simulink subsystem "Init_Frenet_Value"  (R2022b)
settings: Solver=VariableStepAuto  StartTime=0.0  StopTime=10.0  RelTol=1e-3
settings Model: Creator=User  LastModifiedBy=User

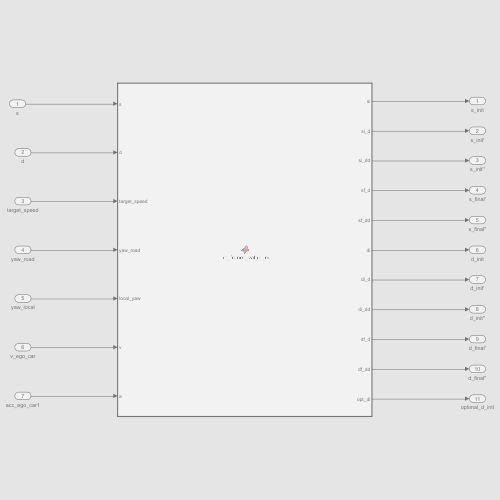
[thumbnail: Simulink's stored preview of the top-level diagram]
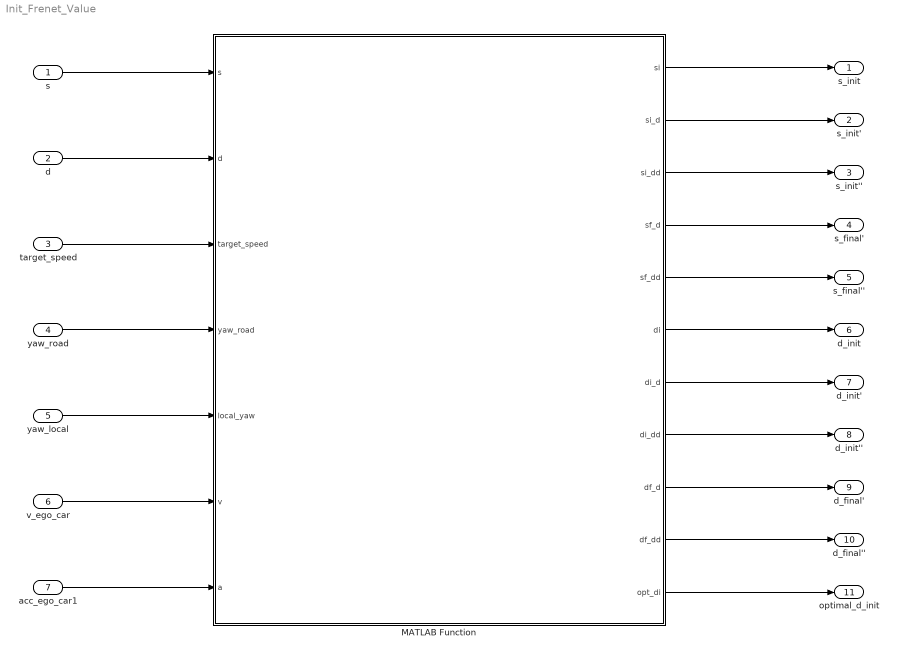
== system Init_Frenet_Value ==
  s : Inport
  d : Inport  Port=2
  target_speed : Inport  Port=3
  yaw_road : Inport  Port=4
  yaw_local : Inport  Port=5
  v_ego_car : Inport  Port=6
  acc_ego_car1 : Inport  Port=7
  MATLAB Function : MATLAB Function  TreatAsAtomicUnit=on
  s_init : Outport
  s_init' : Outport  Port=2
  s_init'' : Outport  Port=3
  s_final' : Outport  Port=4
  s_final'' : Outport  Port=5
  d_init : Outport  Port=6
  d_init' : Outport  Port=7
  d_init'' : Outport  Port=8
  d_final' : Outport  Port=9
  d_final'' : Outport  Port=10
  optimal_d_init : Outport  Port=11
  wires:
  acc_ego_car1/1 -> MATLAB Function/7(a)
  v_ego_car/1 -> MATLAB Function/6(v)
  yaw_local/1 -> MATLAB Function/5(local_yaw)
  MATLAB Function/11(opt_di) -> optimal_d_init/1
  MATLAB Function/10(df_dd) -> d_final''/1
  MATLAB Function/9(df_d) -> d_final'/1
  MATLAB Function/8(di_dd) -> d_init''/1
  MATLAB Function/7(di_d) -> d_init'/1
  MATLAB Function/6(di) -> d_init/1
  MATLAB Function/5(sf_dd) -> s_final''/1
  MATLAB Function/4(sf_d) -> s_final'/1
  MATLAB Function/3(si_dd) -> s_init''/1
  MATLAB Function/2(si_d) -> s_init'/1
  MATLAB Function/1(si) -> s_init/1
  target_speed/1 -> MATLAB Function/3(target_speed)
  yaw_road/1 -> MATLAB Function/4(yaw_road)
  d/1 -> MATLAB Function/2(d)
  s/1 -> MATLAB Function/1(s)

== matlab function Init_Frenet_Value/MATLAB Function ==
  data: s input; si output; d input; target_speed input; yaw_road input; si_d output; si_dd output; sf_d output; sf_dd output; di output; di_d output; di_dd output; df_d output; df_dd output; opt_di output; local_yaw input; v input; a input
function [si, si_d, si_dd, sf_d, sf_dd, di, di_d, di_dd,df_d,df_dd, opt_di] = init_frenet_value_m(s, d, target_speed, yaw_road, local_yaw, v, a)
    [si, si_d, si_dd, sf_d, sf_dd, di, di_d, di_dd,df_d,df_dd, opt_di] = init_frenet_value(s, d, target_speed, yaw_road, local_yaw, v, a);
    
end
